simulink model "aerodynamic_force"  (R2020b)
settings: Solver=FixedStepAuto  StartTime=0.0  StopTime=10.0  RelTol=1e-3
undefined symbols (not defined in the file): C_rho_air, P_A_front_rocket, P_Cd_rocket
settings Model: Creator=Nicolai  LastModifiedBy=Nicolai

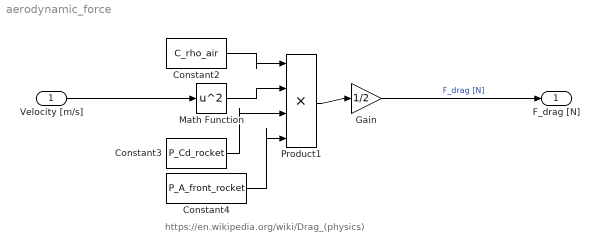
== system aerodynamic_force ==
  note: https://en.wikipedia.org/wiki/Drag_(physics)
  Velocity [m/s] : Inport
  Constant2 : Constant  Value=C_rho_air
  Constant3 : Constant  Value=P_Cd_rocket
  Constant4 : Constant  Value=P_A_front_rocket
  Gain : Gain  Gain=1/2
  Math Function : Math  Operator=square  SaturateOnIntegerOverflow=on
  Product1 : Product  Inputs=4
  F_drag [N] : Outport
  wires:
  Velocity [m/s]/1 -> Math Function/1
  Math Function/1 -> Product1/2
  Product1/1 -> Gain/1
  Gain/1 -> F_drag [N]/1  "F_drag [N]"
  Constant3/1 -> Product1/3
  Constant2/1 -> Product1/1
  Constant4/1 -> Product1/4
